simulink model "sim_altimeter"  (R2024b)
settings: Solver=ode4  StartTime=t_0  StopTime=t_f  FixedStep=dt  RelTol=1e-8
settings Model: Creator=yevge  LastModifiedBy=yevge
settings DebuggingCC: AlgebraicLoopMsg=error  CheckMatrixSingularityMsg=error

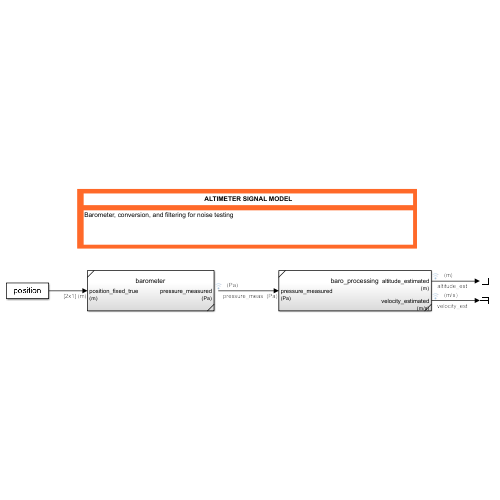
[thumbnail: Simulink's stored preview of the top-level diagram]
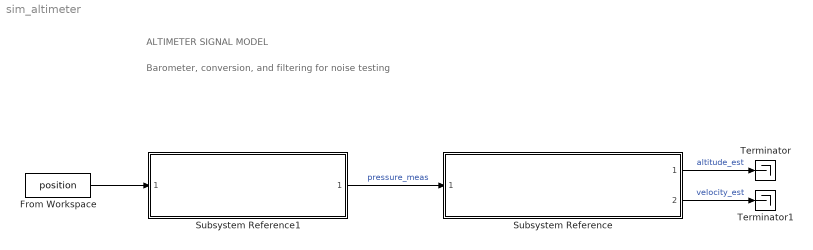
== system sim_altimeter ==
  note: Barometer, conversion, and filtering for noise testing
  note: ALTIMETER SIGNAL MODEL
  From Workspace : FromWorkspace  VariableName=position
  Subsystem Reference : Subsystem  ReferencedSubsystem=baro_processing
  Subsystem Reference1 : Subsystem  ReferencedSubsystem=barometer
  Terminator : Terminator
  Terminator1 : Terminator
  wires:
  Subsystem Reference1/1 -> Subsystem Reference/1  "pressure_meas"
  From Workspace/1 -> Subsystem Reference1/1
  Subsystem Reference/1 -> Terminator/1  "altitude_est"
  Subsystem Reference/2 -> Terminator1/1  "velocity_est"
